simulink model "untitled"  (R2018b)
settings: Solver=VariableStepAuto  StartTime=0.0  StopTime=10.0  RelTol=1e-3
settings Model: Creator=Administrator  LastModifiedBy=Administrator

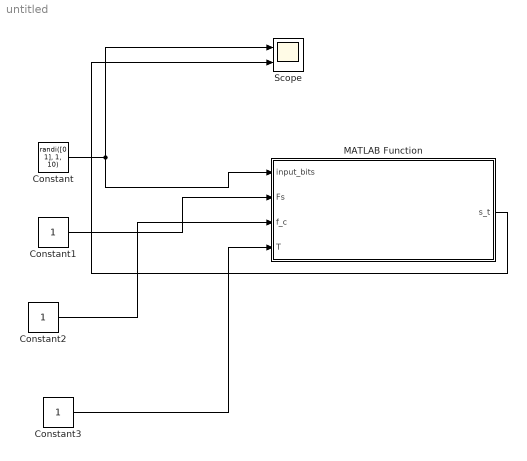
== system untitled ==
  Constant : Constant  Value=randi([0 1], 1, 10)
  Constant1 : Constant
  Constant2 : Constant
  Constant3 : Constant
  MATLAB Function : MATLAB Function  TreatAsAtomicUnit=on
  Scope : Scope  NumInputPorts=2
  wires:
  Constant/1 -> MATLAB Function/1(input_bits), Scope/1
  MATLAB Function/1(s_t) -> Scope/2
  Constant1/1 -> MATLAB Function/2(Fs)
  Constant2/1 -> MATLAB Function/3(f_c)
  Constant3/1 -> MATLAB Function/4(T)

== matlab function untitled/MATLAB Function ==
  data: input_bits input; s_t output [-100000000000..100000000000]; Fs input; f_c input; T input
function s_t = fcn(input_bits, Fs, f_c, T)
    % Function to perform Amplitude Shift Keying (ASK) modulation

    % Number of bits in the input sequence
    num_bits = length(input_bits);  
    
    % Time vector based on the signal duration (duration in seconds)
    t = 0:1/Fs:T-1/Fs;

    % Duration of each bit in time (e.g., 1 ms for 1 kbps bit rate)
    bit_duration = T / num_bits;  
    
    % Initialize the amplitude array for the signal
    A = zeros(1, length(t));
    
    % Map the binary sequence to the amplitude (0 for '0', 1 for '1')
    for i = 1:num_bits
        start_idx = round((i-1) * bit_duration * Fs) + 1;
        end_idx = round(i * bit_duration * Fs);
        A(start_idx:end_idx) = input_bits(i);
    end
    
    % Scale the amplitude (0.5 for '0', 1.0 for '1')
    A_modulated = A * 0.5 + 0.5;
    
    % Generate the ASK modulated signal by multiplying with the carrier wave
    s_t = A_modulated .* cos(2 * pi * f_c * t);  % ASK modulation

    % Explicitly define the output size
    %#codegen
    s_t = reshape(s_t, [1, numel(s_t)]);  % Ensure the output is a fixed-size vector
end
